simulink model "trimfly1"  (Simulink 10.2)
settings: Solver=VariableStepAuto  StartTime=0.0  StopTime=10  RelTol=1e-3
undefined symbols (not defined in the file or in its folder): linsys3
settings Model: Creator=Pro14  LastModifiedBy=Pro14  MultiThreadCoSim=auto
settings DataIOCC: SaveFormat=Dataset  SignalLoggingSaveFormat=Dataset  ReturnWorkspaceOutputs=on
settings OptimizationCC: LifeSpan=auto
settings DebuggingCC: UnderspecifiedInitializationDetection=Simplified  MergeDetectMultiDrivingBlocksExec=error  FcnCallInpInsideContextMsg=error  UnconnectedInputMsg=none  UnconnectedOutputMsg=none  UnconnectedLineMsg=none  SFUnexpectedBacktrackingDiag=error  SFNoUnconditionalDefaultTransitionDiag=error  SFExecutionAtInitializationDiag=warning  ArithmeticOperatorsInVariantConditions=error
settings HardwareCC: ProdBitPerPointer=64  ProdBitPerSizeT=64  ProdBitPerPtrDiffT=64  ProdLargestAtomicFloat=Float  ProdIntDivRoundTo=Zero  ProdEndianess=LittleEndian  ProdWordSize=64  ProdHWDeviceType=Intel->x86-64 (Windows64)
settings ModelReferenceCC: EnableRefExpFcnMdlSchedulingChecks=off  PropagateSignalLabelsOutOfModel=on
settings SFSimCC: SimUseLocalCustomCode=on  CustomCodeUndefinedFunction=FilterOut
settings RTWCC: RTWUseLocalCustomCode=on  GPUComputeCapability=5.0
settings CodeAppCC: StateflowObjectComments=off
settings GRTTargetCC: TargetLangStandard=C99 (ISO)  CombineOutputUpdateFcns=on  GRTInterface=off
settings ConfigComp: CovMetricSettings=dwe  CovSaveCumulativeToWorkspaceVar=off  CovSaveSingleToWorkspaceVar=off  CovExternalEMLEnable=on

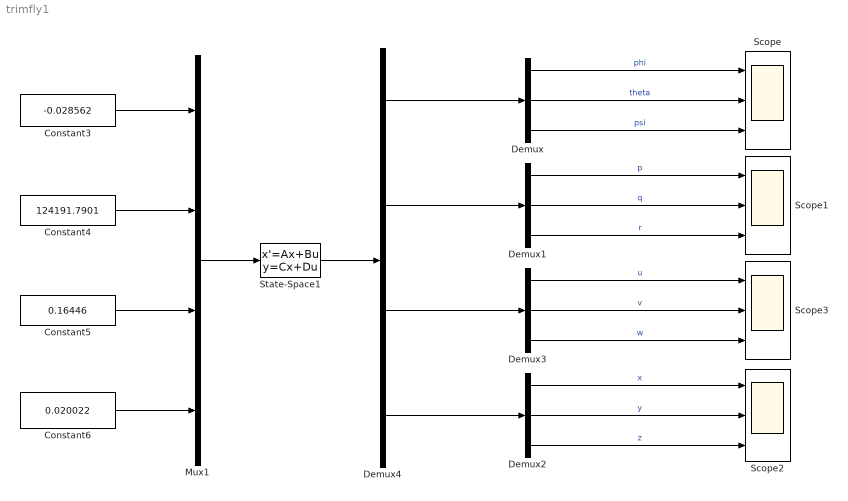
== system trimfly1 ==
  Constant3 : Constant  Value=-0.028562
  Constant4 : Constant  Value=124191.7901
  Constant5 : Constant  Value=0.16446
  Constant6 : Constant  Value=0.020022
  Demux{,1..3} (4 alike) : Demux  Outputs=3
  Demux4 : Demux
  Mux1 : Mux
  Scope{,1..3} (4 alike) : Scope  NumInputPorts=3
  State-Space1 : StateSpace  A=linsys3.A  B=linsys3.B  C=linsys3.C  D=linsys3.D  InitialCondition=[0.029772,0.037541,-0.013252,0,0,0,199.8415,2.8727,7.4235,0,0,-8000]
  wires:
  Constant3/1 -> Mux1/1
  Constant4/1 -> Mux1/2
  Constant5/1 -> Mux1/3
  Constant6/1 -> Mux1/4
  Mux1/1 -> State-Space1/1
  Demux1/3 -> Scope1/3  "r"
  Demux1/1 -> Scope1/1  "p"
  Demux1/2 -> Scope1/2  "q"
  Demux4/3 -> Demux3/1
  Demux3/1 -> Scope3/1  "u"
  Demux2/2 -> Scope2/2  "y"
  Demux4/4 -> Demux2/1
  Demux2/1 -> Scope2/1  "x"
  Demux4/2 -> Demux1/1
  Demux2/3 -> Scope2/3  "z"
  Demux3/2 -> Scope3/2  "v"
  Demux4/1 -> Demux/1
  Demux/2 -> Scope/2  "theta"
  Demux/3 -> Scope/3  "psi"
  Demux/1 -> Scope/1  "phi"
  Demux3/3 -> Scope3/3  "w"
  State-Space1/1 -> Demux4/1
